simulink model "FlottaDroniA_OpenLoop"  (R2025b)
settings: Solver=ode4  StartTime=0.0  StopTime=60  FixedStep=0.01  RelTol=1e-3
libraries: uavutilslib x1
settings Model: Creator=asiabruno  LastModifiedBy=asiabruno
settings DebuggingCC: SFUnusedDataAndEventsDiag=none

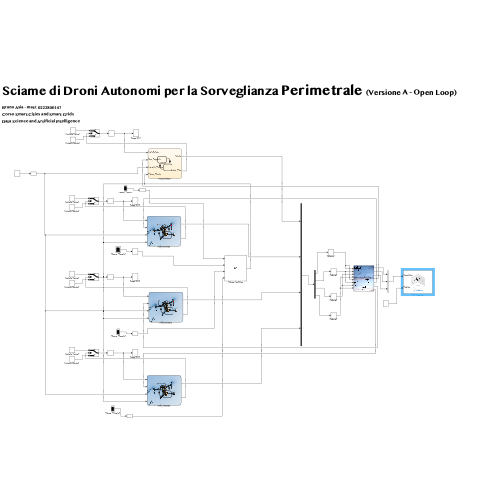
[thumbnail: Simulink's stored preview of the top-level diagram]
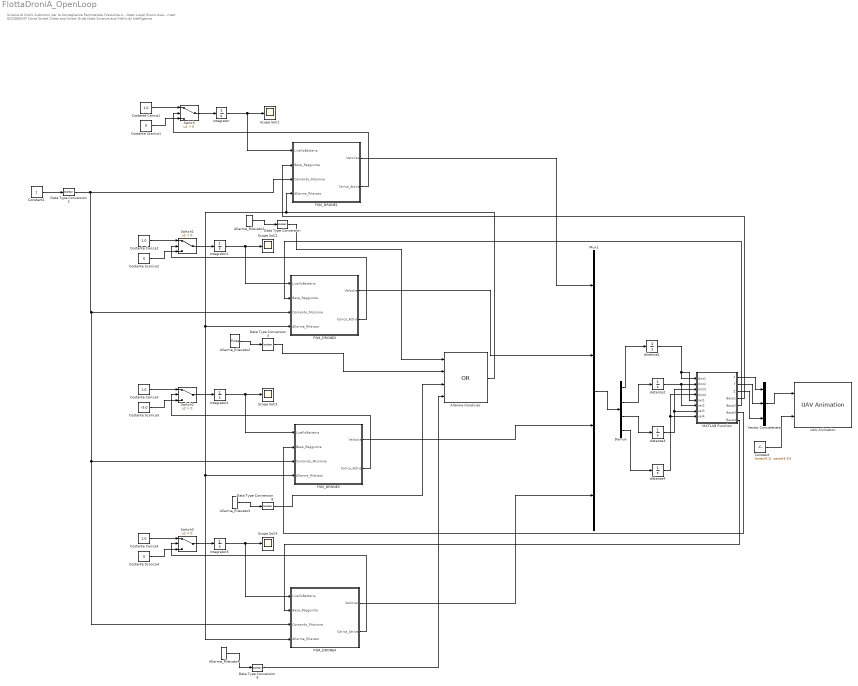
== system FlottaDroniA_OpenLoop ==
  note: Sciame di Droni Autonomi per la Sorveglianza Perimetrale (Versione A - Open Loop)
      | Bruno Asia - matr. 0222800147
      | Corso Smart Cities and Smart Grids
      | Data Science and Artificial Intelligence
  Allarme Condiviso : Logic  Operator=OR  Inputs=4  AllPortsSameDT=off  OutDataTypeStr=boolean
  Allarme_Rilevato{1..4} (4 alike) : DiscretePulseGenerator  PulseType=Time based  Period=1000  PhaseDelay=10
  Constant : Constant  Value=[ones(4,1), zeros(4,3)]
  Constant1 : Constant
  Costante Carica{1..4} (4 alike) : Constant  Value=1.0
  Costante Scarica1 : Constant  Value=0
  Costante Scarica2 : Constant  Value=0
  Costante Scarica3 : Constant  Value=-5.0
  Costante Scarica4 : Constant  Value=0
  Data Type Conversion{,2..3,6,9} (5 alike) : DataTypeConversion  OutDataTypeStr=boolean  SaturateOnIntegerOverflow=off  RndMeth=Floor
  Demux : Demux
  FSM_DRONE1 : Stateflow chart  TreatAsAtomicUnit=on
      settings: PortSchema="{\"entries\":[{\"content\":{\"sides\":[{\"content\":{\"connectorIds\":[\"In1\",\"In3\",\"In4\",\"In2\"]},\"type\":\"ConnectorPlacement.EquallySpacedRectSide\",\"uuid\":\"542c33b0-b79c-4c41-b49d-9733b04c747a\"},{\"content\":{\"connectorIds\":[\"Out1\",\"Out2\"],\"side\":\"RIGHT\"},\"type\":\"ConnectorPlacement.EquallySpacedRectSide\",\"uuid\":\"8da00c1d-9444-4f2d-af6d-9dc6497d2c16\"},{\"content\":{\"side\":\"TOP\"},\"type\":\"ConnectorPlacement.EquallySpacedRectSide\",\"uuid\":\"46ce16a0-96f4-4a94-9b4d-364e0cc1212d\"}]},\"type\":\"ConnectorPlacement.EquallySpacedConnector\",\"uuid\":\"2e9459ac-b079-47ab-be4b-ce2a7ea22f25\"}],\"packageUris\":[\"http://schema.mathworks.com/mf0/Connector/R2020b\"],\"version\":\"1.0\"}"
  FSM_DRONE2 : Stateflow chart  TreatAsAtomicUnit=on
      settings: PortSchema="{\"entries\":[{\"content\":{\"sides\":[{\"content\":{\"connectorIds\":[\"In1\",\"In3\",\"In4\",\"In2\"]},\"type\":\"ConnectorPlacement.EquallySpacedRectSide\",\"uuid\":\"542c33b0-b79c-4c41-b49d-9733b04c747a\"},{\"content\":{\"connectorIds\":[\"Out1\",\"Out2\"],\"side\":\"RIGHT\"},\"type\":\"ConnectorPlacement.EquallySpacedRectSide\",\"uuid\":\"8da00c1d-9444-4f2d-af6d-9dc6497d2c16\"},{\"content\":{\"side\":\"TOP\"},\"type\":\"ConnectorPlacement.EquallySpacedRectSide\",\"uuid\":\"46ce16a0-96f4-4a94-9b4d-364e0cc1212d\"}]},\"type\":\"ConnectorPlacement.EquallySpacedConnector\",\"uuid\":\"2e9459ac-b079-47ab-be4b-ce2a7ea22f25\"}],\"packageUris\":[\"http://schema.mathworks.com/mf0/Connector/R2020b\"],\"version\":\"1.0\"}"
  FSM_DRONE3 : Stateflow chart  TreatAsAtomicUnit=on
      settings: PortSchema="{\"entries\":[{\"content\":{\"sides\":[{\"content\":{\"connectorIds\":[\"In1\",\"In3\",\"In4\",\"In2\"]},\"type\":\"ConnectorPlacement.EquallySpacedRectSide\",\"uuid\":\"542c33b0-b79c-4c41-b49d-9733b04c747a\"},{\"content\":{\"connectorIds\":[\"Out1\",\"Out2\"],\"side\":\"RIGHT\"},\"type\":\"ConnectorPlacement.EquallySpacedRectSide\",\"uuid\":\"8da00c1d-9444-4f2d-af6d-9dc6497d2c16\"},{\"content\":{\"side\":\"TOP\"},\"type\":\"ConnectorPlacement.EquallySpacedRectSide\",\"uuid\":\"46ce16a0-96f4-4a94-9b4d-364e0cc1212d\"},{\"content\":{\"side\":\"BOTTOM\"},\"type\":\"ConnectorPlacement.EquallySpacedRectSide\",\"uuid\":\"b4e8f0de-d973-4b84-b1c9-2233f29a78d7\"}]},\"type\":\"ConnectorPlacement.EquallySpacedConnector\",\"uuid\":\"2e9459ac-b079-47ab-be4b-ce2a7ea22f25\"}],\"packageUris\":[\"http://schema.mathworks.com/mf0/Connector/R2020b\"],\"version\":\"1.0\"}"
  FSM_DRONE4 : Stateflow chart  TreatAsAtomicUnit=on
      settings: PortSchema="{\"entries\":[{\"content\":{\"sides\":[{\"content\":{\"connectorIds\":[\"In1\",\"In3\",\"In4\",\"In2\"]},\"type\":\"ConnectorPlacement.EquallySpacedRectSide\",\"uuid\":\"542c33b0-b79c-4c41-b49d-9733b04c747a\"},{\"content\":{\"connectorIds\":[\"Out1\",\"Out2\"],\"side\":\"RIGHT\"},\"type\":\"ConnectorPlacement.EquallySpacedRectSide\",\"uuid\":\"8da00c1d-9444-4f2d-af6d-9dc6497d2c16\"},{\"content\":{\"side\":\"TOP\"},\"type\":\"ConnectorPlacement.EquallySpacedRectSide\",\"uuid\":\"46ce16a0-96f4-4a94-9b4d-364e0cc1212d\"},{\"content\":{\"side\":\"BOTTOM\"},\"type\":\"ConnectorPlacement.EquallySpacedRectSide\",\"uuid\":\"b9d5a143-2063-4bcd-935e-de4fd80c6cec\"}]},\"type\":\"ConnectorPlacement.EquallySpacedConnector\",\"uuid\":\"2e9459ac-b079-47ab-be4b-ce2a7ea22f25\"}],\"packageUris\":[\"http://schema.mathworks.com/mf0/Connector/R2020b\"],\"version\":\"1.0\"}"
  Integrator{,1..3} (4 alike) : Integrator  InitialCondition=100.0
  MATLAB Function : MATLAB Function  TreatAsAtomicUnit=on
  Mux1 : Mux
  Scope SoC{1..4} (4 alike) : Scope
      Scope SoC1 settings: ActiveDisplayYMinimum=-16.596275958902623  ActiveDisplayYMaximum=180.09726991892936
      Scope SoC2 settings: ActiveDisplayYMinimum=-16.596275958902623  ActiveDisplayYMaximum=180.09726991892936  DataLoggingVariableName=ScopeData2
      Scope SoC3 settings: ActiveDisplayYMinimum=-16.596275958902623  ActiveDisplayYMaximum=180.09726991892936  DataLoggingVariableName=ScopeData3
      Scope SoC4 settings: ActiveDisplayYMinimum=-16.596275958902623  ActiveDisplayYMaximum=180.09726991892936  DataLoggingVariableName=ScopeData4
  Switch{,1..3} (4 alike) : Switch  Criteria=u2 > Threshold  SaturateOnIntegerOverflow=off  InputSameDT=off
  UAV Animation : uavutilslib/UAV Animation  NumUAV=4  DynamicUAVConfig=off  UAVType=Multirotor  UAVSize=8  UAVColor=[1 0 0]  UAVTrajectoryAlpha=1  InertialZDirection=Up  RotationFormat=Quaternion  DrawMarkers=off  SampleTime=-1
  Vector Concatenate : Concatenate  NumInputs=3  Mode=Multidimensional array  ConcatenateDimension=2
  distanza{1..4} (4 alike) : Integrator
  wires:
  Costante Carica1/1 -> Switch/1
  Costante Scarica1/1 -> Switch/3
  Switch/1 -> Integrator/1
  Integrator/1 -> Scope SoC1/1, FSM_DRONE1/1(LivelloBatteria)
  Allarme_Rilevato1/1 -> Data Type Conversion/1
  Data Type Conversion/1 -> Allarme Condiviso/1
  Constant1/1 -> Data Type Conversion2/1
  Data Type Conversion2/1 -> FSM_DRONE1/4(Comando_Missione), FSM_DRONE4/4(Comando_Missione), FSM_DRONE3/4(Comando_Missione), FSM_DRONE2/4(Comando_Missione)
  Allarme_Rilevato2/1 -> Data Type Conversion3/1
  Integrator1/1 -> Scope SoC2/1, FSM_DRONE2/1(LivelloBatteria)
  Costante Scarica2/1 -> Switch1/3
  Switch1/1 -> Integrator1/1
  Data Type Conversion3/1 -> Allarme Condiviso/2
  Costante Carica2/1 -> Switch1/1
  Allarme_Rilevato3/1 -> Data Type Conversion6/1
  Integrator2/1 -> Scope SoC3/1, FSM_DRONE3/1(LivelloBatteria)
  Costante Scarica3/1 -> Switch2/3
  Switch2/1 -> Integrator2/1
  Data Type Conversion6/1 -> Allarme Condiviso/3
  Costante Carica3/1 -> Switch2/1
  Allarme_Rilevato4/1 -> Data Type Conversion9/1
  Integrator3/1 -> Scope SoC4/1, FSM_DRONE4/1(LivelloBatteria)
  Costante Scarica4/1 -> Switch3/3
  Switch3/1 -> Integrator3/1
  Data Type Conversion9/1 -> Allarme Condiviso/4
  Costante Carica4/1 -> Switch3/1
  FSM_DRONE1/1(Velocita) -> Mux1/1
  FSM_DRONE2/1(Velocita) -> Mux1/2
  FSM_DRONE3/1(Velocita) -> Mux1/3
  FSM_DRONE4/1(Velocita) -> Mux1/4
  Allarme Condiviso/1 -> FSM_DRONE3/2(Allarme_Rilevato), FSM_DRONE4/2(Allarme_Rilevato), FSM_DRONE2/2(Allarme_Rilevato), FSM_DRONE1/2(Allarme_Rilevato)
  FSM_DRONE1/2(Carica_Attiva) -> Switch/2
  FSM_DRONE2/2(Carica_Attiva) -> Switch1/2
  FSM_DRONE3/2(Carica_Attiva) -> Switch2/2
  FSM_DRONE4/2(Carica_Attiva) -> Switch3/2
  Mux1/1 -> Demux/1
  Demux/1 -> distanza1/1
  Demux/2 -> distanza2/1
  Demux/3 -> distanza3/1
  Demux/4 -> distanza4/1
  distanza1/1 -> MATLAB Function/5(vel1), MATLAB Function/1(dist1)
  distanza2/1 -> MATLAB Function/6(vel2), MATLAB Function/2(dist2)
  distanza3/1 -> MATLAB Function/3(dist3), MATLAB Function/7(vel3)
  distanza4/1 -> MATLAB Function/4(dist4), MATLAB Function/8(vel4)
  MATLAB Function/1(X) -> Vector Concatenate/1
  MATLAB Function/2(Y) -> Vector Concatenate/2
  MATLAB Function/3(Z) -> Vector Concatenate/3
  Vector Concatenate/1 -> UAV Animation/1
  Constant/1 -> UAV Animation/2
  MATLAB Function/4(Base1) -> FSM_DRONE1/3(Base_Raggiunta)
  MATLAB Function/5(Base2) -> FSM_DRONE2/3(Base_Raggiunta)
  MATLAB Function/6(Base3) -> FSM_DRONE3/3(Base_Raggiunta)
  MATLAB Function/7(Base4) -> FSM_DRONE4/3(Base_Raggiunta)

== stateflow chart FlottaDroniA_OpenLoop/FSM_DRONE4 ==
  state IDLE_LOOKING
    entry: Velocita = 0; Carica_Attiva = logical(1);
  state PATROL
    entry: Velocita = 5.0; Carica_Attiva = logical(0);
  state INVESTIGATE
    entry: Velocita = 2.0; Carica_Attiva = logical(0);
  state RETURN_TO_BASE
    entry: Velocita = 8.0; Carica_Attiva = logical(0);
  (default) -> IDLE_LOOKING
  IDLE_LOOKING -> PATROL : [LivelloBatteria >= 90 ]
  RETURN_TO_BASE -> IDLE_LOOKING : [Base_Raggiunta > 0.5]
  PATROL -> RETURN_TO_BASE [order 1] : [LivelloBatteria <= 30]
  INVESTIGATE -> PATROL [order 2] : after(5, sec)
  PATROL -> INVESTIGATE [order 2] : [Allarme_Rilevato]
  INVESTIGATE -> RETURN_TO_BASE [order 1] : [LivelloBatteria <= 10]
  data: LivelloBatteria input double; Allarme_Rilevato input boolean; Base_Raggiunta input double; Comando_Missione input boolean; Velocita output double; Carica_Attiva output boolean; SoC_Ready constant double =90; SoC_Return constant double =30; T_invest constant double =5; SoC_Critical constant double =10; V_return constant double; V_patrol constant double; V_invest constant double; TY_BASE constant double; TX_BASE constant double
  data LivelloBatteria settings: description=feedback dell integrator per la decisione sulla batteria
  data Allarme_Rilevato settings: description=viene dal pulse generator (delay = 50s)
  data Base_Raggiunta settings: description=viene dallo step (fine missione)
  data Comando_Missione settings: description=viene da pulse generator (delay = 0s)
  data Velocita settings: description=va al mux per scope output

== matlab function FlottaDroniA_OpenLoop/MATLAB Function ==
  settings: updateMethod=DISCRETE  sampleTime=0.1
  data: dist1 input; X output; dist2 input; dist3 input; dist4 input; Y output; Z output; vel1 input; vel2 input; vel3 input; vel4 input; Base1 output double; Base2 output double; Base3 output double; Base4 output double
function [X, Y, Z, Base1, Base2, Base3, Base4] = fcn(dist1, dist2, dist3, dist4, vel1, vel2, vel3, vel4)

    LATO = 100.0;
    ALT = 10.0;
    
    dists = [dist1; dist2; dist3; dist4];
    vels = [vel1; vel2; vel3; vel4];
    
    X = zeros(4,1);
    Y = zeros(4,1);
    Z = ones(4,1) * ALT;
    BaseRaggiunta_out = zeros(4,1); 

    for i = 1:4
        
        % --- 1. Calcolo Posizione di Pattugliamento ---
        percorso_doppio = 2 * LATO;
        dist_mod = mod(dists(i), percorso_doppio);
        pos_pattuglia = 0.0;
        
        if dist_mod < LATO
            pos_pattuglia = dist_mod;
        else
            pos_pattuglia = percorso_doppio - dist_mod;
        end
        
        X_patt = 0.0; Y_patt = 0.0;
        if i == 1
            X_patt = pos_pattuglia; Y_patt = 0;
        elseif i == 2
            X_patt = LATO; Y_patt = pos_pattuglia;
        elseif i == 3
            X_patt = LATO - pos_pattuglia; Y_patt = LATO;
        elseif i == 4
            X_patt = 0; Y_patt = LATO - pos_pattuglia;
        end
        
        
        % --- 2. Decisione Posizione  ---
        
        if vels(i) == 0.0
            % STATO: IDLE (V=0.0)
            % Il drone è arrivato e DEVE rimanere sulle coordinate [0,0]
            X(i) = 0.0;
            Y(i) = 0.0;
            BaseRaggiunta_out(i) = 1.0; 
        
        elseif vels(i) == 8.0
            % STATO: RETURN_TO_BASE (V=8.0)
            % Il drone sta TORNANDO. NON è ancora arrivato.
            
            % il rientro è più veloce 
            
            X(i) = X_patt;
            Y(i) = Y_patt;
            
            % Controlla se il drone è arrivato 
            if X(i) < 1 && Y(i) < 1
                 BaseRaggiunta_out(i) = 1.0; 
            end

        else 
            % STATO: PATROL (V=5.0) o INVESTIGATE (V=2.0)
            X(i) = X_patt;
            Y(i) = Y_patt;
            BaseRaggiunta_out(i) = 0.0; 
        end
    end
    
    % --- 3. Assegna Uscite ---
    Base1 = BaseRaggiunta_out(1);
    Base2 = BaseRaggiunta_out(2);
    Base3 = BaseRaggiunta_out(3);
    Base4 = BaseRaggiunta_out(4);
end

== stateflow chart FlottaDroniA_OpenLoop/FSM_DRONE1 ==
  state IDLE_LOOKING
    entry: Velocita = 0; Carica_Attiva = logical(1);
  state PATROL
    entry: Velocita = 5.0; Carica_Attiva = logical(0);
  state INVESTIGATE
    entry: Velocita = 2.0; Carica_Attiva = logical(0);
  state RETURN_TO_BASE
    entry: Velocita = 8.0; Carica_Attiva = logical(0);
  (default) -> IDLE_LOOKING
  IDLE_LOOKING -> PATROL : [LivelloBatteria >= 90 ]
  RETURN_TO_BASE -> IDLE_LOOKING : [Base_Raggiunta > 0.5]
  PATROL -> RETURN_TO_BASE [order 1] : [LivelloBatteria <= 30]
  INVESTIGATE -> PATROL [order 2] : after(5, sec)
  PATROL -> INVESTIGATE [order 2] : [Allarme_Rilevato]
  INVESTIGATE -> RETURN_TO_BASE [order 1] : [LivelloBatteria <= 10]
  data: LivelloBatteria input double; Allarme_Rilevato input boolean; Base_Raggiunta input double; Comando_Missione input boolean; Velocita output double; Carica_Attiva output boolean; SoC_Ready constant double =90; SoC_Return constant double =30; T_invest constant double =5; SoC_Critical constant double =10; V_return constant double; V_patrol constant double; V_invest constant double; TY_BASE constant double; TX_BASE constant double
  data LivelloBatteria settings: description=feedback dell integrator per la decisione sulla batteria
  data Allarme_Rilevato settings: description=viene dal pulse generator (delay = 50s)
  data Base_Raggiunta settings: description=viene dallo step (fine missione)
  data Comando_Missione settings: description=viene da pulse generator (delay = 0s)
  data Velocita settings: description=va al mux per scope output

== stateflow chart FlottaDroniA_OpenLoop/FSM_DRONE2 ==
  state IDLE_LOOKING
    entry: Velocita = 0; Carica_Attiva = logical(1);
  state PATROL
    entry: Velocita = 5.0; Carica_Attiva = logical(0);
  state INVESTIGATE
    entry: Velocita = 2.0; Carica_Attiva = logical(0);
  state RETURN_TO_BASE
    entry: Velocita = 8.0; Carica_Attiva = logical(0);
  (default) -> IDLE_LOOKING
  IDLE_LOOKING -> PATROL : [LivelloBatteria >= 90 ]
  RETURN_TO_BASE -> IDLE_LOOKING : [Base_Raggiunta > 0.5]
  PATROL -> RETURN_TO_BASE [order 1] : [LivelloBatteria <= 30]
  INVESTIGATE -> PATROL [order 2] : after(5, sec)
  PATROL -> INVESTIGATE [order 2] : [Allarme_Rilevato]
  INVESTIGATE -> RETURN_TO_BASE [order 1] : [LivelloBatteria <= 10]
  data: LivelloBatteria input double; Allarme_Rilevato input boolean; Base_Raggiunta input double; Comando_Missione input boolean; Velocita output double; Carica_Attiva output boolean; SoC_Ready constant double =90; SoC_Return constant double =30; T_invest constant double =5; SoC_Critical constant double =10; V_return constant double; V_patrol constant double; V_invest constant double; TY_BASE constant double; TX_BASE constant double
  data LivelloBatteria settings: description=feedback dell integrator per la decisione sulla batteria
  data Allarme_Rilevato settings: description=viene dal pulse generator (delay = 50s)
  data Base_Raggiunta settings: description=viene dallo step (fine missione)
  data Comando_Missione settings: description=viene da pulse generator (delay = 0s)
  data Velocita settings: description=va al mux per scope output

== stateflow chart FlottaDroniA_OpenLoop/FSM_DRONE3 ==
  state IDLE_LOOKING
    entry: Velocita = 0; Carica_Attiva = logical(1);
  state PATROL
    entry: Velocita = 5.0; Carica_Attiva = logical(0);
  state INVESTIGATE
    entry: Velocita = 2.0; Carica_Attiva = logical(0);
  state RETURN_TO_BASE
    entry: Velocita = 8.0; Carica_Attiva = logical(0);
  (default) -> IDLE_LOOKING
  IDLE_LOOKING -> PATROL : [LivelloBatteria >= 90]
  RETURN_TO_BASE -> IDLE_LOOKING : [Base_Raggiunta > 0.5]
  PATROL -> RETURN_TO_BASE [order 1] : [LivelloBatteria <= 30]
  INVESTIGATE -> PATROL [order 2] : after(5, sec)
  PATROL -> INVESTIGATE [order 2] : [Allarme_Rilevato]
  INVESTIGATE -> RETURN_TO_BASE [order 1] : [LivelloBatteria <= 10]
  data: LivelloBatteria input double; Allarme_Rilevato input boolean; Base_Raggiunta input double; Comando_Missione input boolean; Velocita output double; Carica_Attiva output boolean; SoC_Ready constant double =90; SoC_Return constant double =30; T_invest constant double =5; SoC_Critical constant double =10; V_return constant double; V_patrol constant double; V_invest constant double; TY_BASE constant double; TX_BASE constant double
  data LivelloBatteria settings: description=feedback dell integrator per la decisione sulla batteria
  data Allarme_Rilevato settings: description=viene dal pulse generator (delay = 50s)
  data Base_Raggiunta settings: description=viene dallo step (fine missione)
  data Comando_Missione settings: description=viene da pulse generator (delay = 0s)
  data Velocita settings: description=va al mux per scope output
